simulink model "f4"  (R2021b)
settings: Solver=VariableStepAuto  StartTime=0.0  StopTime=10.0  RelTol=1e-3
settings Model: Creator=asus  LastModifiedBy=asus

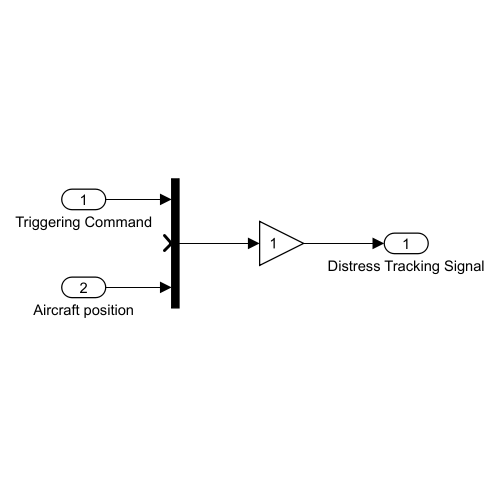
[thumbnail: Simulink's stored preview of the top-level diagram]
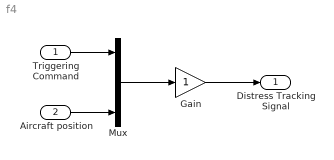
== system f4 ==
  Triggering Command : Inport
  Aircraft position : Inport  Port=2
  Gain : Gain
  Mux : Mux  Inputs=3
  Distress Tracking Signal : Outport
  wires:
  Gain/1 -> Distress Tracking Signal/1
  Triggering Command/1 -> Mux/1
  Aircraft position/1 -> Mux/3
  Mux/1 -> Gain/1
